simulink model "task_3d"  (R2014b)
settings: Solver=ode45  StartTime=0.0  StopTime=450  RelTol=1e-3
values from neighbouring files (symbols this model uses):
  A = [-0.322 0.052 0.028 -1.12 0.002 ... (first row only)    [parameters.m]
  B = [0 0 0 0 10]'    [parameters.m]
  C = [0 0 0 1 ... (first row only)    [parameters.m]
  g = 9.81    [parameters.m]
  Kd_phi = 2.15    [parameters.m]
  Ki_chi = 0.1954    [parameters.m]
  Kp_chi = 3.7547    [parameters.m]
  Kp_phi = -5/3    (= -1.66666666667)    [parameters.m]
  Vg = 637/3.6    (= 176.944444444)    [parameters.m]
settings Model: Creator=sondr_000  LastModifiedBy=Ultrawack
settings OptimizationCC: BlockReduction=off  BooleanDataType=off  UseDivisionForNetSlopeComputation=off  SimCompilerOptimization=off
settings DebuggingCC: SaveWithParameterizedLinksMsg=none  UnderspecifiedInitializationDetection=Classic  MergeDetectMultiDrivingBlocksExec=none  SignalResolutionControl=TryResolveAllWithWarning  SolverPrmCheckMsg=none  FcnCallInpInsideContextMsg=error  FrameProcessingCompatibilityMsg=error  SFExecutionAtInitializationDiag=none
settings HardwareCC: ProdBitPerSizeT=32  ProdBitPerPtrDiffT=32  TargetUnknown=on
settings RTWCC: RTWCompilerOptimization=off
settings ConfigComp: CovMetricSettings=dw  CovHtmlReporting=on  CovSaveCumulativeToWorkspaceVar=on  CovSaveSingleToWorkspaceVar=on  CovExternalEMLEnable=off  CovSFcnEnable=off

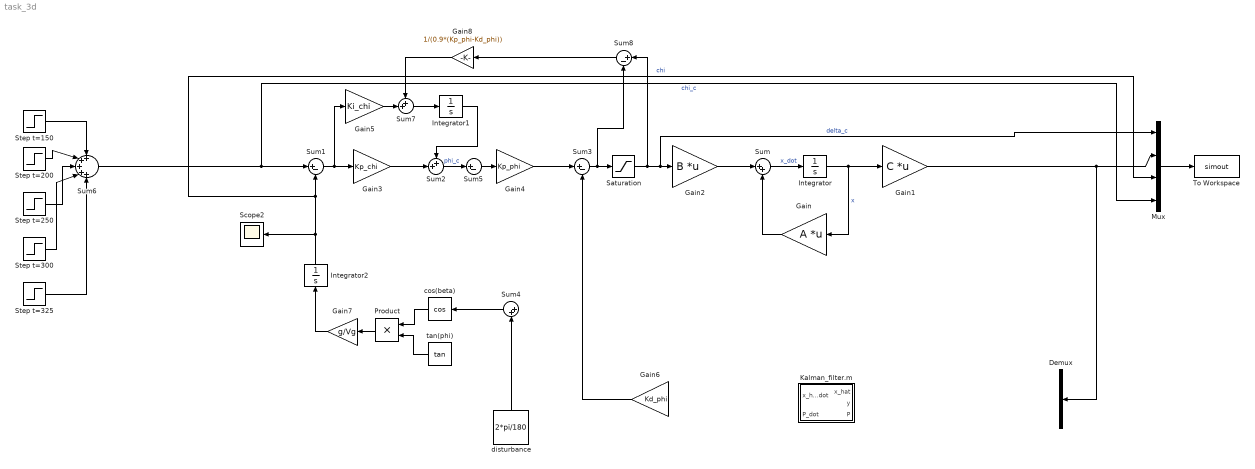
== system task_3d ==
  Demux : Demux  Outputs=3
  Gain : Gain  Gain=A  Multiplication=Matrix(K*u)
  Gain1 : Gain  Gain=C  Multiplication=Matrix(K*u)
  Gain2 : Gain  Gain=B  Multiplication=Matrix(K*u)
  Gain3 : Gain  Gain=Kp_chi
  Gain4 : Gain  Gain=Kp_phi
  Gain5 : Gain  Gain=Ki_chi
  Gain6 : Gain  Gain=Kd_phi
  Gain7 : Gain  Gain=g/Vg
  Gain8 : Gain  Gain=1/(0.9*(Kp_phi-Kd_phi))
  Integrator : Integrator
  Integrator1 : Integrator
  Integrator2 : Integrator
  Kalman_filter.m : MATLAB Function  TreatAsAtomicUnit=on
  Mux : Mux
  Product : Product
  Saturation : Saturate  UpperLimit=25*pi/180  LowerLimit=-025*pi/180
  Scope2 : Scope
      settings: YMin=-0.11374  YMax=1.02365  SaveName=ScopeData2
  Step t=150 : Step  Time=100  After=0.20  SampleTime=0
  Step t=200 : Step  Time=200  After=0.15  SampleTime=0
  Step t=250 : Step  Time=220  After=0.20  SampleTime=0
  Step t=300 : Step  Time=300  After=0.25  SampleTime=0
  Step t=325 : Step  Time=375  After=-0.10  SampleTime=0
  Sum : Sum  Inputs=|++
  Sum{1,3,5,8} (4 alike) : Sum  Inputs=|+-
  Sum2 : Sum  Inputs=++|
  Sum4 : Sum  Inputs=|++
  Sum6 : Sum  Inputs=+++++
  Sum7 : Sum  Inputs=++|
  To Workspace : ToWorkspace  VariableName=simout  SaveFormat=Timeseries  SampleTime=-1
  cos(beta) : Trigonometry  Operator=cos
  disturbance : Constant  Value=2*pi/180
  tan(phi) : Trigonometry  Operator=tan
  wires:
  Gain1/1 -> Mux/2, Demux/1
  Integrator/1 -> Gain/1, Gain1/1  "x"
  Sum/1 -> Integrator/1  "x_dot"
  Gain/1 -> Sum/2
  Gain2/1 -> Sum/1
  Saturation/1 -> Sum8/1, Mux/1, Gain2/1  "delta_c"
  Sum1/1 -> Gain5/1, Gain3/1
  Sum3/1 -> Sum8/2, Saturation/1
  Gain4/1 -> Sum3/1
  Gain6/1 -> Sum3/2
  Sum6/1 -> Sum1/1, Mux/4  "chi_c"
  Gain3/1 -> Sum2/2
  Sum5/1 -> Gain4/1
  Sum2/1 -> Sum5/1  "phi_c"
  Mux/1 -> To Workspace/1
  Integrator2/1 -> Scope2/1, Mux/3, Sum1/2  "chi"
  Gain7/1 -> Integrator2/1
  tan(phi)/1 -> Product/2
  cos(beta)/1 -> Product/1
  Product/1 -> Gain7/1
  Sum4/1 -> cos(beta)/1
  disturbance/1 -> Sum4/2
  Step t=150/1 -> Sum6/1
  Step t=200/1 -> Sum6/2
  Step t=250/1 -> Sum6/3
  Step t=300/1 -> Sum6/4
  Step t=325/1 -> Sum6/5
  Integrator1/1 -> Sum2/1
  Sum7/1 -> Integrator1/1
  Gain5/1 -> Sum7/2
  Sum8/1 -> Gain8/1
  Gain8/1 -> Sum7/1

== matlab function task_3d/Kalman_filter.m ==
  data: x_hat input; y input; P input; x_hat_dot output; P_dot output
function [ x_hat_dot, P_dot ] = Kalman_filter( x_hat, y, P )
K = P*C'\R;
x_hat_dot = A*x_hat + B*u + K*(y - C*x_hat);
P_dot = A*P + P*A' + E*Q*E' - P*H'\R*H*P;
end
